simulink model "Regelstrecke_EinAusgangsLinearisierung_2024b"  (R2024b)
settings: Solver=VariableStepAuto  StartTime=0.0  StopTime=10
InitFcn:
  | % Definition der Konstanten
  | k  = 1.380649e-23;
  | e  = 1.602176634e-19;
  | T0 = 273.15; % absoluter Nullpunkt in K
  | T_C = 25; % Temperatur in °C
  | UT = k * (T0 + T_C) / e;
  | IS = 1e-8;
  | R  = 1e3;
  | L  = 100e-3;
  | C1 = 100e-9;
  | C2 = 1e-6;
  | 
  | % Werte der Stellgrößen
  | I0 = 10e-3;
  | U0 = 12;
  | 
  | syms U1_val U2_val IL_val U0_val I0_val
  | x = [U1_val, U2_val, IL_val];
  | %Zerlegung in System-, Ausgangs- und Eingangswirkung
  | f_ea = [
  |     -IS*exp(-U2_val/UT)/C1 + IL_val/C1;
  |     IL_val/C2;
  |     -U1_val/L - U2_val/L - R*IL_val/L
  | ]
  | g_ea = [
  |     0, 0;
  |     0, -1/C2;
  |     1/L, 0;
  | ]
  | g_ea_U0 = [
  |     0;
  |     0;
  |     1/L;
  | ]
  | g_ea_I0 = [
  |     0;
  |     -I0/C2;
  |     0;
  | ]
  | h_ea = U2_val %for y = xi set h_ea at position i to 1
  | 
  | %Lie-Ableitungen berechnen
  | Lf = h_ea;
  | Lf_h = Lf;
  | r = 0;
  | 
  | Lf_r = sym(zeros(10,1))
  | Lf_r(1) = Lf_h
  | 
  | 
  | while true
  |     LgLf = jacobian(Lf, x) * g_ea % x = [U1; U2; IL]
  |     if LgLf ~= 0
  |         % vermutlich notwendig, um L_f^r h anstelle von L_f^{(r-1)} h zu
  |         % erhalten
  |         Lf = jacobian(Lf, x) * f_ea
  |         Lf_h = Lf
  |         %
  |         break;
  |     end
  |     Lf = jacobian(Lf, x) * f_ea % x = [U1; U2; IL], Lf = IL/C2
  |     Lf_h = Lf
  |     Lf_r(r+2) = Lf_h
  |     r = r + 1
  | end
  | 
  | r = r + 1
  | 
  | phi = Lf_r
  | disp(Lf_r)
  | 
  | syms v
  | L_nom = v - Lf_h % letzte Lf
  | L_denom = LgLf
  | %L = L_nom * pinv(L_denom)
  | 
  | L_pinv = pinv(L_denom)
  | 
  | alpha = LgLf
  | beta = Lf_h
  | 
  | 
  | 
  | %%%A-, B-, und C-Matrix
  | A = zeros(r);
  | for i=1:r
  |     for j=1:r
  |         if j == i+1
  |             A(i,j) = 1;
  |         end
  |     end
  | end
  | 
  | %%Oder:
  | %A = diag(ones(r-1,1), 1);
  | 
  | B = zeros(r,1);
  | B(r) = 1
  | 
  | C = zeros(1,r)
  | C(1) = 1
  | 
  | %syms U2_ref Kp
  | %v = Kp * (U2_ref - U2);
  | 
  | p = [-20, -2-2j, -2+2j];
  | 
  | G = place(A, B, p)
settings Model: Creator=richa  LastModifiedBy=richa
settings ConfigComp: CovBoundaryAbsTol=1.0e-5

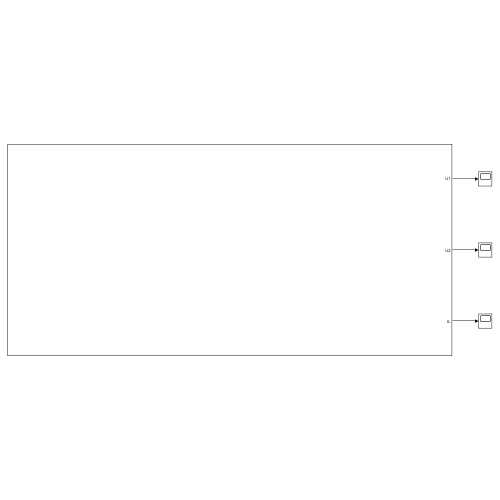
[thumbnail: Simulink's stored preview of the top-level diagram]
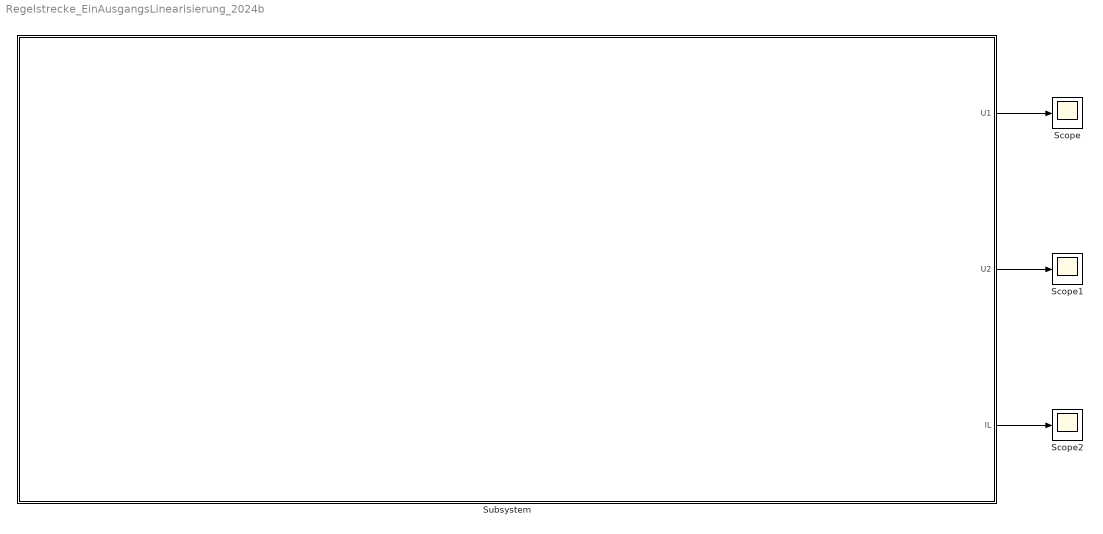
== system Regelstrecke_EinAusgangsLinearisierung_2024b ==
  Scope : Scope
  Scope1 : Scope
  Scope2 : Scope
  Subsystem : Subsystem
  wires:
  Subsystem/1(U1) -> Scope/1
  Subsystem/2(U2) -> Scope1/1
  Subsystem/3(IL) -> Scope2/1

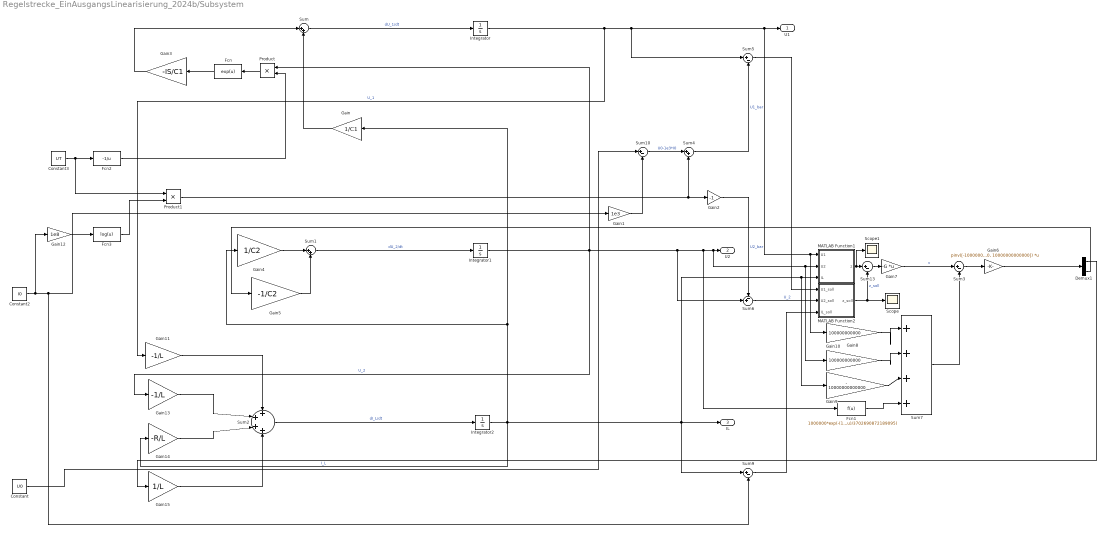
== system Regelstrecke_EinAusgangsLinearisierung_2024b/Subsystem ==
  Constant : Constant  Value=U0
  Constant2 : Constant  Value=I0
  Constant3 : Constant  Value=UT
  Demux1 : Demux  Outputs=2
  Fcn : Fcn  Expr=exp(u)
  Fcn1 : Fcn  Expr=1000000*exp(-(144115188075855872*u)/3702690872189095)
  Fcn2 : Fcn  Expr=-1/u
  Fcn3 : Fcn  Expr=log(u)
  Gain : Gain  Gain=1/C1
  Gain1 : Gain  Gain=1e3
  Gain10 : Gain  Gain=100000000000
  Gain11 : Gain  Gain=-1/L
  Gain12 : Gain  Gain=1e8
  Gain13 : Gain  Gain=-1/L
  Gain14 : Gain  Gain=-R/L
  Gain15 : Gain  Gain=1/L
  Gain2 : Gain  Gain=-1
  Gain3 : Gain  Gain=-IS/C1
  Gain4 : Gain  Gain=1/C2
  Gain5 : Gain  Gain=-1/C2
  Gain6 : Gain  Gain=pinv([-100000000000, 10000000000000])  Multiplication=Matrix(K*u)
  Gain7 : Gain  Gain=-G  Multiplication=Matrix(K*u)
  Gain8 : Gain  Gain=100000000000
  Gain9 : Gain  Gain=- 10000000000000
  Integrator : Integrator
  Integrator1 : Integrator
  Integrator2 : Integrator
  MATLAB Function1 : MATLAB Function  TreatAsAtomicUnit=on
  MATLAB Function2 : MATLAB Function  TreatAsAtomicUnit=on
  Product : Product
  Product1 : Product
  Scope : Scope
  Scope1 : Scope
  Sum : Sum  Inputs=|++
  Sum1 : Sum  Inputs=|++
  Sum{3,5,9..10,13} (5 alike) : Sum  Inputs=|+-
  Sum2 : Sum  Inputs=++++
  Sum4 : Sum  Inputs=|++
  Sum6 : Sum  Inputs=-+|
  Sum7 : Sum  Inputs=|++++
  U1 : Outport
  U2 : Outport  Port=2
  IL : Outport  Port=3
  wires:
  Gain7/1 -> Sum3/1  "v"
  Sum3/1 -> Gain6/1
  Gain8/1 -> Sum7/1
  Sum7/1 -> Sum3/2
  Gain9/1 -> Sum7/3
  Gain10/1 -> Sum7/2
  Fcn1/1 -> Sum7/4
  Gain6/1 -> Demux1/1
  Fcn3/1 -> Product1/2
  Gain4/1 -> Sum1/1
  Gain11/1 -> Sum2/1
  Constant/1 -> Sum10/1
  Fcn2/1 -> Product/2
  Gain/1 -> Sum/2
  Gain1/1 -> Sum10/2
  Gain12/1 -> Fcn3/1
  Gain13/1 -> Sum2/2
  Gain5/1 -> Sum1/2
  Integrator1/1 -> Fcn1/1, Gain10/1, MATLAB Function1/2(U2), U2/1, Sum6/2, Product/1, Gain13/1  "U_2"
  Gain3/1 -> Sum/1
  Sum1/1 -> Integrator1/1  "dU_2/dt"
  Sum4/1 -> Sum5/2  "U1_bar"
  Constant2/1 -> Gain12/1, Gain1/1, Sum9/2
  Integrator/1 -> Gain8/1, MATLAB Function1/1(U1), U1/1, Sum5/1, Gain11/1  "U_1"
  Constant3/1 -> Product1/1, Fcn2/1
  Product/1 -> Fcn/1
  Gain14/1 -> Sum2/3
  Product1/1 -> Gain2/1, Sum4/2
  Sum/1 -> Integrator/1  "dU_1/dt"
  Sum10/1 -> Sum4/1  "U0-1e3*I0"
  Fcn/1 -> Gain3/1
  Gain15/1 -> Sum2/4
  Sum2/1 -> Integrator2/1  "dI_L/dt"
  Integrator2/1 -> Sum9/1, Gain9/1, MATLAB Function1/3(IL), IL/1, Gain14/1, Gain/1, Gain4/1  "I_L"
  Gain2/1 -> Sum6/1  "U2_bar"
  Sum5/1 -> MATLAB Function2/1(U1_soll)
  Sum6/1 -> MATLAB Function2/2(U2_soll)  "U_2"
  Sum9/1 -> MATLAB Function2/3(IL_soll)
  Sum13/1 -> Gain7/1
  MATLAB Function1/1(z) -> Scope1/1, Sum13/1
  MATLAB Function2/1(z_soll) -> Scope/1, Sum13/2  "z_soll"
  Demux1/1 -> Gain15/1
  Demux1/2 -> Gain5/1

== matlab function Regelstrecke_EinAusgangsLinearisierung_2024b/Subsystem/MATLAB Function2 ==
  data: U1_soll input; z_soll output; U2_soll input; IL_soll input
function z_soll = fcn(U1_soll, U2_soll, IL_soll)
    z_soll = [U2_soll; 1000000*IL_soll; -10000000000*IL_soll - 10000000*U1_soll - 10000000*U2_soll];
end

== matlab function Regelstrecke_EinAusgangsLinearisierung_2024b/Subsystem/MATLAB Function1 ==
  data: U1 input; z output; U2 input; IL input
function z = fcn(U1, U2, IL)
    z = [U2; 1000000*IL; -10000000000*IL - 10000000*U1 - 10000000*U2];
end
